simulink model "Simple_4Quad_payload_04"  (R2018b)
settings: Solver=VariableStepAuto  StartTime=0.0  StopTime=60  RelTol=1e-3
InitFcn:
  | Simple_4Quad_payload_04_const
values from neighbouring files (symbols this model uses):
  All_rho = [d1 0 0 ... (first row only)    [Colab_4Quad_model_01_const.m]    (also in Colab_4Quad_model_02_const.m; Simple_4Quad_payload_04_const.m; Simple_4Quad_payload_05_const.m; Simple_4Quad_payload_06_const.m)
  B_ob = [zeros(3);eye(3)]    [Simple_4Quad_payload_04_const.m]    (also in Simple_4Quad_payload_05_const.m; Simple_4Quad_payload_06_const.m; Simple_4Quad_payload_07_const.m; Simple_4Quad_payload_08_const.m)
  BBT_inv = ((B'*B)^(-1))*B'    [Simple_2Quad_payload_03_const.m]    (also in Simple_4Quad_payload_04_const.m = ((BR'*BR)^(-1))*BR'; Simple_4Quad_payload_05_const.m = ((BR'*BR)^(-1))*BR'; Simple_4Quad_payload_06_const.m = ((BR'*BR)^(-1))*BR'; Simple_4Quad_payload_07_const.m = ((BR'*BR)^(-1))*BR')
  BR = 1e0*eye(n)    [Simple_4Quad_payload_04_const.m]    (also in Simple_4Quad_payload_05_const.m; Simple_4Quad_payload_06_const.m; Simple_4Quad_payload_07_const.m; Simple_4Quad_payload_08_const.m)
  C_ob = [eye(3) zeros(3)]    [Simple_4Quad_payload_04_const.m]    (also in Simple_4Quad_payload_05_const.m; Simple_4Quad_payload_06_const.m; Simple_4Quad_payload_07_const.m; Simple_4Quad_payload_08_const.m)
  d1 = 0.25    [Colab_4Quad_model_01_const.m]    (also in Colab_4Quad_model_02_const.m = 0.5; Simple_4Quad_payload_01_const.m = 1; Simple_4Quad_payload_02_const.m = 1; Simple_4Quad_payload_03_const.m = 1)
  d2 = 0.25    [Colab_4Quad_model_01_const.m]    (also in Colab_4Quad_model_02_const.m = 0.5; Simple_4Quad_payload_01_const.m = 1; Simple_4Quad_payload_02_const.m = 1; Simple_4Quad_payload_03_const.m = 1)
  Des_rel_dist = 2    [Simple_4Quad_payload_01_const.m]    (also in Simple_4Quad_payload_02_const.m = 4; Simple_4Quad_payload_03_const.m = 4; Simple_4Quad_payload_04_const.m; Simple_4Quad_payload_05_const.m)
  g = 9.81    [Colab_4Quad_model_01_const.m]    (also in Colab_4Quad_model_02_const.m; Simple_2Quad_payload_01_const.m; Simple_2Quad_payload_02_const.m; Simple_2Quad_payload_03_const.m)
  gamma_0 = 1e-0*diag([1e-3;1e-0])    [Simple_2Quad_payload_03_const.m]    (also in Simple_4Quad_payload_04_const.m = 1e-0*diag([1e-6*ones(3,1);1e-0*ones(3,1)]); Simple_4Quad_payload_05_const.m = 1e-1*diag([1e-6*ones(3,1);1e-0*ones(3,1)]); Simple_4Quad_payload_06_const.m = 1e-0*diag([1e-6*ones(3,1);1e-0*ones(3,1)]); Simple_4Quad_payload_07_const.m = 1e-0*diag([1e-6*ones(3,1);1e-0*ones(3,1)]))
  gamma_1 = 1e+2*diag([1e-3;1e-0])    [Simple_2Quad_payload_03_const.m]    (also in Simple_4Quad_payload_04_const.m = 1e+2*diag([1e-6*ones(3,1);1e-0*ones(3,1)]); Simple_4Quad_payload_05_const.m = 1e+2*diag([1e-6*ones(3,1);1e-0*ones(3,1)]); Simple_4Quad_payload_06_const.m = 1e+3*diag([1e-6*ones(3,1);1e-0*ones(3,1)]); Simple_4Quad_payload_07_const.m = 1e+3*diag([1e-6*ones(3,1);1e-0*ones(3,1)]))
  Ix = 0.166667    [Colab_4Quad_model_01_const.m]    (also in Colab_4Quad_model_02_const.m = 0.02; Simple_4Quad_payload_01_const.m = 1; Simple_4Quad_payload_02_const.m = 1; Simple_4Quad_payload_03_const.m = 1)
  Iy = 0.166667    [Colab_4Quad_model_01_const.m]    (also in Colab_4Quad_model_02_const.m = 0.02; Simple_4Quad_payload_01_const.m = 1; Simple_4Quad_payload_02_const.m = 1; Simple_4Quad_payload_03_const.m = 1)
  Iz = 0.166667    [Colab_4Quad_model_01_const.m]    (also in Colab_4Quad_model_02_const.m = 0.02; Simple_4Quad_payload_01_const.m = 1; Simple_4Quad_payload_02_const.m = 1; Simple_4Quad_payload_03_const.m = 1)
  Jo = diag([Ix;Iy;Iz])    [Colab_4Quad_model_01_const.m]    (also in Colab_4Quad_model_02_const.m; Simple_4Quad_payload_04_const.m; Simple_4Quad_payload_05_const.m; Simple_4Quad_payload_06_const.m)
  Jq = diag([0.0291 0.0291 0.0552])    [Colab_4Quad_model_01_const.m]    (also in Colab_4Quad_model_02_const.m = diag([0.03 0.03 0.06]); Simple_4Quad_payload_03_const.m = 1.2416e-3 * diag([1 1 2]); Simple_4Quad_payload_04_const.m = 1 * diag([1 1 2]); Simple_4Quad_payload_05_const.m = 1 * diag([1 1 2]))
  k1 = 1    [Simple_2Quad_payload_03_const.m]    (also in Simple_4Quad_payload_04_const.m; Simple_4Quad_payload_05_const.m; Simple_4Quad_payload_06_const.m; Simple_4Quad_payload_07_const.m)
  k2 = 0.1    [Simple_2Quad_payload_03_const.m]    (also in Simple_4Quad_payload_04_const.m; Simple_4Quad_payload_05_const.m; Simple_4Quad_payload_06_const.m; Simple_4Quad_payload_07_const.m)
  ki1_N = 0    [Simple_4Quad_payload_02_const.m]    (also in Simple_4Quad_payload_03_const.m; Simple_4Quad_payload_04_const.m; Simple_4Quad_payload_05_const.m; Simple_4Quad_payload_06_const.m)
  ki1_S = 0    [Simple_4Quad_payload_02_const.m]    (also in Simple_4Quad_payload_03_const.m; Simple_4Quad_payload_04_const.m)
  ki2_N = 0    [Simple_4Quad_payload_02_const.m]    (also in Simple_4Quad_payload_03_const.m; Simple_4Quad_payload_04_const.m; Simple_4Quad_payload_05_const.m; Simple_4Quad_payload_06_const.m = 10)
  ki2_S = 0    [Simple_4Quad_payload_02_const.m]    (also in Simple_4Quad_payload_03_const.m; Simple_4Quad_payload_04_const.m)
  kp1_N = 10    [Simple_4Quad_payload_02_const.m]    (also in Simple_4Quad_payload_03_const.m; Simple_4Quad_payload_04_const.m; Simple_4Quad_payload_05_const.m = 1; Simple_4Quad_payload_06_const.m = 1)
  kp1_S = 10    [Simple_4Quad_payload_02_const.m]    (also in Simple_4Quad_payload_03_const.m; Simple_4Quad_payload_04_const.m)
  kp2_N = 100    [Simple_4Quad_payload_02_const.m]    (also in Simple_4Quad_payload_03_const.m; Simple_4Quad_payload_04_const.m; Simple_4Quad_payload_05_const.m = 1; Simple_4Quad_payload_06_const.m = 1)
  kp2_S = 100    [Simple_4Quad_payload_02_const.m]    (also in Simple_4Quad_payload_03_const.m; Simple_4Quad_payload_04_const.m)
  l = 3.1819    [Colab_4Quad_model_01_const.m]    (also in Colab_4Quad_model_02_const.m = 3; Simple_2Quad_payload_04_const.m = 1; Simple_4Quad_payload_01_const.m = 1; Simple_4Quad_payload_02_const.m = 2)
  m = 1.5    [Colab_4Quad_model_01_const.m]    (also in Colab_4Quad_model_02_const.m; Simple_2Quad_payload_04_const.m = 1; Simple_4Quad_payload_01_const.m = 1; Simple_4Quad_payload_02_const.m = 1)
  M = 1.0    (= 1)    [Colab_4Quad_model_01_const.m]    (also in Colab_4Quad_model_02_const.m; Simple_2Quad_payload_01_const.m; Simple_2Quad_payload_02_const.m; Simple_2Quad_payload_03_const.m)
  Md = 1*[1;1;1]    [Simple_2Quad_payload_04_const.m]    (also in Simple_4Quad_payload_01_const.m = 1*[1;1;1;1;1;1]; Simple_4Quad_payload_02_const.m = 1*[1;1;1;1;1;1]; Simple_4Quad_payload_03_const.m = 1*[1;1;1;1;1;1]; Simple_4Quad_payload_04_const.m = 1*[1;1;1;1;1;1])
  n = 2    [Simple_2Quad_payload_03_const.m]    (also in Simple_4Quad_payload_03_const.m = 6; Simple_4Quad_payload_04_const.m = 6; Simple_4Quad_payload_05_const.m = 6; Simple_4Quad_payload_06_const.m = 6)
  Q_ob = var_u_ob * eye(6)    [Simple_4Quad_payload_04_const.m]    (also in Simple_4Quad_payload_05_const.m; Simple_4Quad_payload_06_const.m; Simple_4Quad_payload_07_const.m; Simple_4Quad_payload_08_const.m)
  QR = 1e-0*eye(n)    [Simple_4Quad_payload_04_const.m]    (also in Simple_4Quad_payload_05_const.m = 1e-1*eye(n); Simple_4Quad_payload_06_const.m; Simple_4Quad_payload_07_const.m; Simple_4Quad_payload_08_const.m)
  R = 1e+0*eye(n)    [Simple_2Quad_payload_03_const.m]    (also in Simple_4Quad_payload_04_const.m = 1e+0*eye(m); Simple_4Quad_payload_05_const.m = 1e+0*eye(m); Simple_4Quad_payload_06_const.m; Simple_4Quad_payload_07_const.m)
  R_ob = var_y_ob * eye(3)    [Simple_4Quad_payload_04_const.m]    (also in Simple_4Quad_payload_05_const.m; Simple_4Quad_payload_06_const.m; Simple_4Quad_payload_07_const.m; Simple_4Quad_payload_08_const.m)
  rho_0 = 1e-0    (= 1)    [Simple_2Quad_payload_03_const.m]    (also in Simple_4Quad_payload_04_const.m; Simple_4Quad_payload_05_const.m = 0.1; Simple_4Quad_payload_06_const.m; Simple_4Quad_payload_07_const.m)
  rho_1 = 1e-0    (= 1)    [Simple_2Quad_payload_03_const.m]    (also in Simple_4Quad_payload_04_const.m; Simple_4Quad_payload_05_const.m; Simple_4Quad_payload_06_const.m; Simple_4Quad_payload_07_const.m)
libraries: simulink x16
(part 1 of 4)
settings Model: Creator=ali  LastModifiedBy=asafae

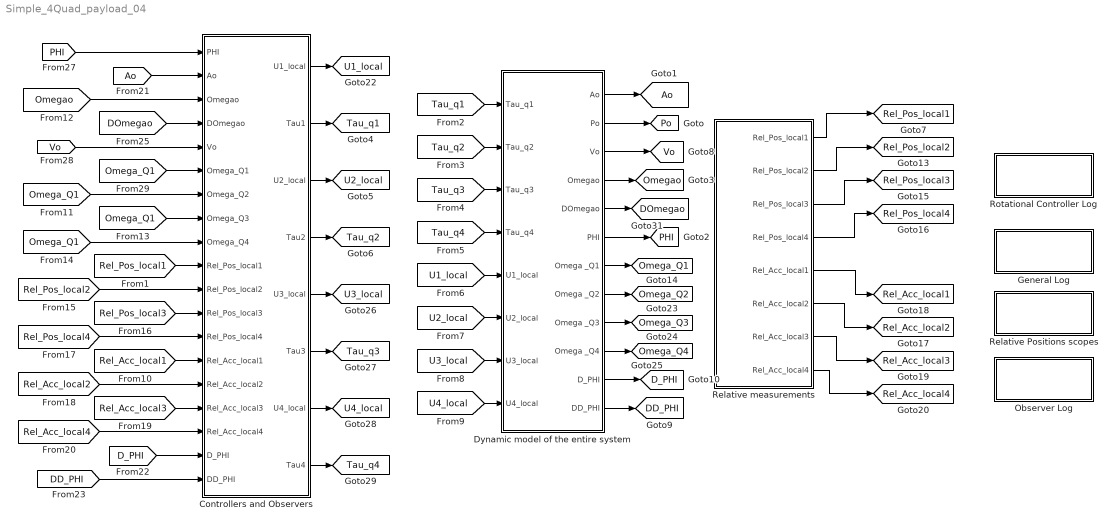
== system Simple_4Quad_payload_04 ==
  Controllers and Observers : Subsystem
  Dynamic model of the entire system : Subsystem
  General Log : Subsystem
  Observer Log : Subsystem
  Relative Positions scopes : Subsystem
  Relative measurements : Subsystem
  Rotational Controller Log : Subsystem
  tag scope: Ao=global, DD_PHI=global, DOmegao=global, D_PHI=global, Omega_Q1=global, Omega_Q2=global, Omega_Q3=global, Omega_Q4=global, Omegao=global, PHI=global, Po=global, Rel_Acc_local1=global, Rel_Acc_local2=global, Rel_Acc_local3=global, Rel_Acc_local4=global, Rel_Pos_local1=global, Rel_Pos_local2=global, Rel_Pos_local3=global, Rel_Pos_local4=global, Tau_q1=global, Tau_q2=global, Tau_q3=global, Tau_q4=global, U1_local=global, U2_local=global, U3_local=global, U4_local=global, Vo=global
  wires:
  [Tau_q1] -> Dynamic model of the entire system/1(Tau_q1)
  [Tau_q2] -> Dynamic model of the entire system/2(Tau_q2)
  [Tau_q3] -> Dynamic model of the entire system/3(Tau_q3)
  [Tau_q4] -> Dynamic model of the entire system/4(Tau_q4)
  [U1_local] -> Dynamic model of the entire system/5(U1_local)
  [U2_local] -> Dynamic model of the entire system/6(U2_local)
  [U3_local] -> Dynamic model of the entire system/7(U3_local)
  [U4_local] -> Dynamic model of the entire system/8(U4_local)
  Dynamic model of the entire system/6(PHI) -> [PHI]
  Dynamic model of the entire system/4(Omegao) -> [Omegao]
  Dynamic model of the entire system/1(Ao) -> [Ao]
  Dynamic model of the entire system/2(Po) -> [Po]
  Dynamic model of the entire system/5(DOmegao) -> [DOmegao]
  Dynamic model of the entire system/7(Omega _Q1) -> [Omega_Q1]
  Dynamic model of the entire system/8(Omega _Q2) -> [Omega_Q2]
  Dynamic model of the entire system/9(Omega _Q3) -> [Omega_Q3]
  Dynamic model of the entire system/10(Omega _Q4) -> [Omega_Q4]
  Controllers and Observers/1(U1_local) -> [U1_local]
  Controllers and Observers/2(Tau1) -> [Tau_q1]
  Controllers and Observers/3(U2_local) -> [U2_local]
  Controllers and Observers/4(Tau2) -> [Tau_q2]
  Controllers and Observers/8(Tau4) -> [Tau_q4]
  Controllers and Observers/7(U4_local) -> [U4_local]
  Controllers and Observers/6(Tau3) -> [Tau_q3]
  Controllers and Observers/5(U3_local) -> [U3_local]
  [Omegao] -> Controllers and Observers/3(Omegao)
  [DOmegao] -> Controllers and Observers/4(DOmegao)
  [Omega_Q1] -> Controllers and Observers/6(Omega_Q1)
  [Omega_Q1] -> Controllers and Observers/7(Omega_Q2)
  [Omega_Q1] -> Controllers and Observers/8(Omega_Q3)
  [Omega_Q1] -> Controllers and Observers/9(Omega_Q4)
  [Rel_Pos_local1] -> Controllers and Observers/10(Rel_Pos_local1)
  [Rel_Pos_local2] -> Controllers and Observers/11(Rel_Pos_local2)
  [Rel_Pos_local3] -> Controllers and Observers/12(Rel_Pos_local3)
  [Rel_Pos_local4] -> Controllers and Observers/13(Rel_Pos_local4)
  [Rel_Acc_local1] -> Controllers and Observers/14(Rel_Acc_local1)
  [Rel_Acc_local2] -> Controllers and Observers/15(Rel_Acc_local2)
  [Rel_Acc_local3] -> Controllers and Observers/16(Rel_Acc_local3)
  [Rel_Acc_local4] -> Controllers and Observers/17(Rel_Acc_local4)
  Relative measurements/1(Rel_Pos_local1) -> [Rel_Pos_local1]
  Relative measurements/2(Rel_Pos_local2) -> [Rel_Pos_local2]
  Relative measurements/3(Rel_Pos_local3) -> [Rel_Pos_local3]
  Relative measurements/4(Rel_Pos_local4) -> [Rel_Pos_local4]
  Relative measurements/5(Rel_Acc_local1) -> [Rel_Acc_local1]
  Relative measurements/6(Rel_Acc_local2) -> [Rel_Acc_local2]
  Relative measurements/7(Rel_Acc_local3) -> [Rel_Acc_local3]
  Relative measurements/8(Rel_Acc_local4) -> [Rel_Acc_local4]
  Dynamic model of the entire system/3(Vo) -> [Vo]
  [Vo] -> Controllers and Observers/5(Vo)
  [PHI] -> Controllers and Observers/1(PHI)
  [Ao] -> Controllers and Observers/2(Ao)
  Dynamic model of the entire system/11(D_PHI) -> [D_PHI]
  Dynamic model of the entire system/12(DD_PHI) -> [DD_PHI]
  [D_PHI] -> Controllers and Observers/18(D_PHI)
  [DD_PHI] -> Controllers and Observers/19(DD_PHI)

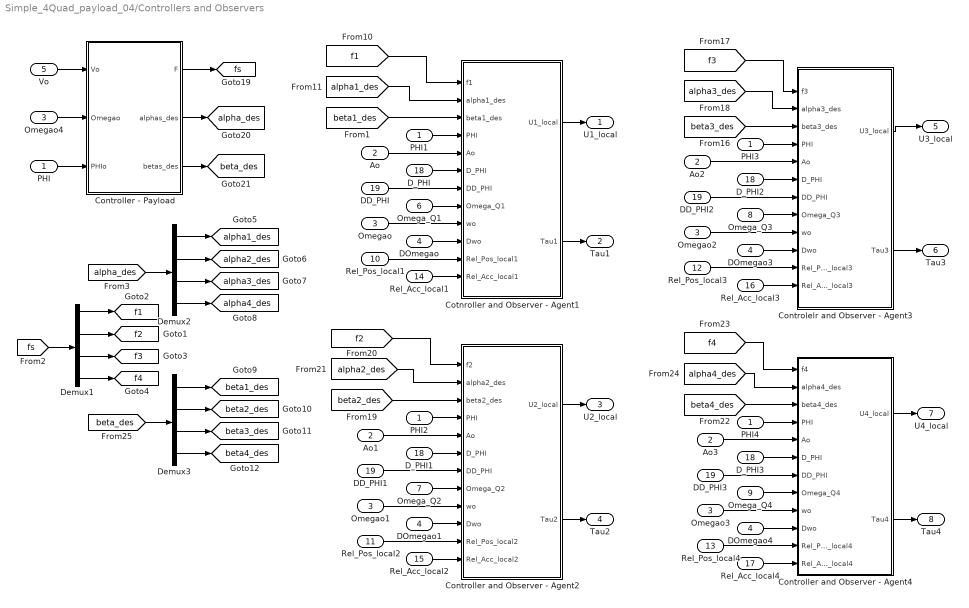
== system Simple_4Quad_payload_04/Controllers and Observers ==
  PHI : Inport
  Ao : Inport  Port=2
  Omegao : Inport  Port=3
  DOmegao : Inport  Port=4
  Vo : Inport  Port=5
  Omega_Q1 : Inport  Port=6
  Omega_Q2 : Inport  Port=7
  Omega_Q3 : Inport  Port=8
  Omega_Q4 : Inport  Port=9
  Rel_Pos_local1 : Inport  Port=10
  Rel_Pos_local2 : Inport  Port=11
  Rel_Pos_local3 : Inport  Port=12
  Rel_Pos_local4 : Inport  Port=13
  Rel_Acc_local1 : Inport  Port=14
  Rel_Acc_local2 : Inport  Port=15
  Rel_Acc_local3 : Inport  Port=16
  Rel_Acc_local4 : Inport  Port=17
  D_PHI : Inport  Port=18
  DD_PHI : Inport  Port=19
  Ao1 : InportShadow  Port=2
  Ao2 : InportShadow  Port=2
  Ao3 : InportShadow  Port=2
  Controlelr and Observer - Agent3 : Subsystem
  Controller - Payload : Subsystem
  Controller and Observer - Agent2 : Subsystem
  Controller and Observer - Agent4 : Subsystem
  "Cotnroller and Observer - Agent1 " : Subsystem
  DD_PHI1 : InportShadow  Port=19
  DD_PHI2 : InportShadow  Port=19
  DD_PHI3 : InportShadow  Port=19
  DOmegao1 : InportShadow  Port=4
  DOmegao3 : InportShadow  Port=4
  DOmegao4 : InportShadow  Port=4
  D_PHI1 : InportShadow  Port=18
  D_PHI2 : InportShadow  Port=18
  D_PHI3 : InportShadow  Port=18
  Demux1 : Demux
  Demux2 : Demux
  Demux3 : Demux
  Omegao{1..4} (4 alike) : InportShadow  Port=3
  PHI{1..4} (4 alike) : InportShadow
  U1_local : Outport
  Tau1 : Outport  Port=2
  U2_local : Outport  Port=3
  Tau2 : Outport  Port=4
  U3_local : Outport  Port=5
  Tau3 : Outport  Port=6
  U4_local : Outport  Port=7
  Tau4 : Outport  Port=8
  tag scope: alpha1_des=global, alpha2_des=global, alpha3_des=global, alpha4_des=global, alpha_des=global, beta1_des=global, beta2_des=global, beta3_des=global, beta4_des=global, beta_des=global, f1=global, f2=global, f3=global, f4=global, fs=global
  wires:
  Controller and Observer - Agent4/2(Tau4) -> Tau4/1
  Controller and Observer - Agent4/1(U4_local) -> U4_local/1
  Controlelr and Observer - Agent3/2(Tau3) -> Tau3/1
  Controlelr and Observer - Agent3/1(U3_local) -> U3_local/1
  Controller and Observer - Agent2/1(U2_local) -> U2_local/1
  "Cotnroller and Observer - Agent1 "/1(U1_local) -> U1_local/1
  Controller and Observer - Agent2/2(Tau2) -> Tau2/1
  Omega_Q1/1 -> "Cotnroller and Observer - Agent1 "/8(Omega_Q1)
  Omega_Q3/1 -> Controlelr and Observer - Agent3/8(Omega_Q3)
  Omega_Q4/1 -> Controller and Observer - Agent4/8(Omega_Q4)
  Omega_Q2/1 -> Controller and Observer - Agent2/8(Omega_Q2)
  "Cotnroller and Observer - Agent1 "/2(Tau1) -> Tau1/1
  [f1] -> "Cotnroller and Observer - Agent1 "/1(f1)
  Controller - Payload/2(alphas_des) -> [alpha_des]
  Vo/1 -> Controller - Payload/1(Vo)
  Omegao4/1 -> Controller - Payload/2(Omegao)
  PHI/1 -> Controller - Payload/3(PHIo)
  Controller - Payload/1(F) -> [fs]
  Controller - Payload/3(betas_des) -> [beta_des]
  [beta1_des] -> "Cotnroller and Observer - Agent1 "/3(beta1_des)
  [alpha1_des] -> "Cotnroller and Observer - Agent1 "/2(alpha1_des)
  Rel_Pos_local1/1 -> "Cotnroller and Observer - Agent1 "/11(Rel_Pos_local1)
  Rel_Acc_local1/1 -> "Cotnroller and Observer - Agent1 "/12(Rel_Acc_local1)
  Rel_Pos_local2/1 -> Controller and Observer - Agent2/11(Rel_Pos_local2)
  Rel_Acc_local2/1 -> Controller and Observer - Agent2/12(Rel_Acc_local2)
  Rel_Pos_local4/1 -> Controller and Observer - Agent4/11(Rel_Pos_local4)
  Rel_Acc_local4/1 -> Controller and Observer - Agent4/12(Rel_Acc_local4)
  Rel_Pos_local3/1 -> Controlelr and Observer - Agent3/11(Rel_Pos_local3)
  Rel_Acc_local3/1 -> Controlelr and Observer - Agent3/12(Rel_Acc_local3)
  [f3] -> Controlelr and Observer - Agent3/1(f3)
  [alpha3_des] -> Controlelr and Observer - Agent3/2(alpha3_des)
  [beta3_des] -> Controlelr and Observer - Agent3/3(beta3_des)
  [f2] -> Controller and Observer - Agent2/1(f2)
  [alpha2_des] -> Controller and Observer - Agent2/2(alpha2_des)
  [beta2_des] -> Controller and Observer - Agent2/3(beta2_des)
  [f4] -> Controller and Observer - Agent4/1(f4)
  [alpha4_des] -> Controller and Observer - Agent4/2(alpha4_des)
  [beta4_des] -> Controller and Observer - Agent4/3(beta4_des)
  DOmegao/1 -> "Cotnroller and Observer - Agent1 "/10(Dwo)
  DOmegao1/1 -> Controller and Observer - Agent2/10(Dwo)
  DOmegao3/1 -> Controlelr and Observer - Agent3/10(Dwo)
  DOmegao4/1 -> Controller and Observer - Agent4/10(Dwo)
  Omegao/1 -> "Cotnroller and Observer - Agent1 "/9(wo)
  Omegao2/1 -> Controlelr and Observer - Agent3/9(wo)
  Omegao1/1 -> Controller and Observer - Agent2/9(wo)
  Omegao3/1 -> Controller and Observer - Agent4/9(wo)
  Demux2/2 -> [alpha2_des]
  Demux3/3 -> [beta3_des]
  Demux2/4 -> [alpha4_des]
  Demux2/3 -> [alpha3_des]
  Demux1/4 -> [f4]
  Demux2/1 -> [alpha1_des]
  Demux1/1 -> [f1]
  [alpha_des] -> Demux2/1
  Demux3/4 -> [beta4_des]
  [beta_des] -> Demux3/1
  [fs] -> Demux1/1
  Demux3/2 -> [beta2_des]
  Demux1/3 -> [f3]
  Demux1/2 -> [f2]
  Demux3/1 -> [beta1_des]
  PHI1/1 -> "Cotnroller and Observer - Agent1 "/4(PHI)
  Ao/1 -> "Cotnroller and Observer - Agent1 "/5(Ao)
  PHI2/1 -> Controller and Observer - Agent2/4(PHI)
  Ao1/1 -> Controller and Observer - Agent2/5(Ao)
  PHI3/1 -> Controlelr and Observer - Agent3/4(PHI)
  Ao2/1 -> Controlelr and Observer - Agent3/5(Ao)
  PHI4/1 -> Controller and Observer - Agent4/4(PHI)
  Ao3/1 -> Controller and Observer - Agent4/5(Ao)
  D_PHI/1 -> "Cotnroller and Observer - Agent1 "/6(D_PHI)
  DD_PHI/1 -> "Cotnroller and Observer - Agent1 "/7(DD_PHI)
  DD_PHI1/1 -> Controller and Observer - Agent2/7(DD_PHI)
  D_PHI1/1 -> Controller and Observer - Agent2/6(D_PHI)
  D_PHI2/1 -> Controlelr and Observer - Agent3/6(D_PHI)
  DD_PHI2/1 -> Controlelr and Observer - Agent3/7(DD_PHI)
  D_PHI3/1 -> Controller and Observer - Agent4/6(D_PHI)
  DD_PHI3/1 -> Controller and Observer - Agent4/7(DD_PHI)

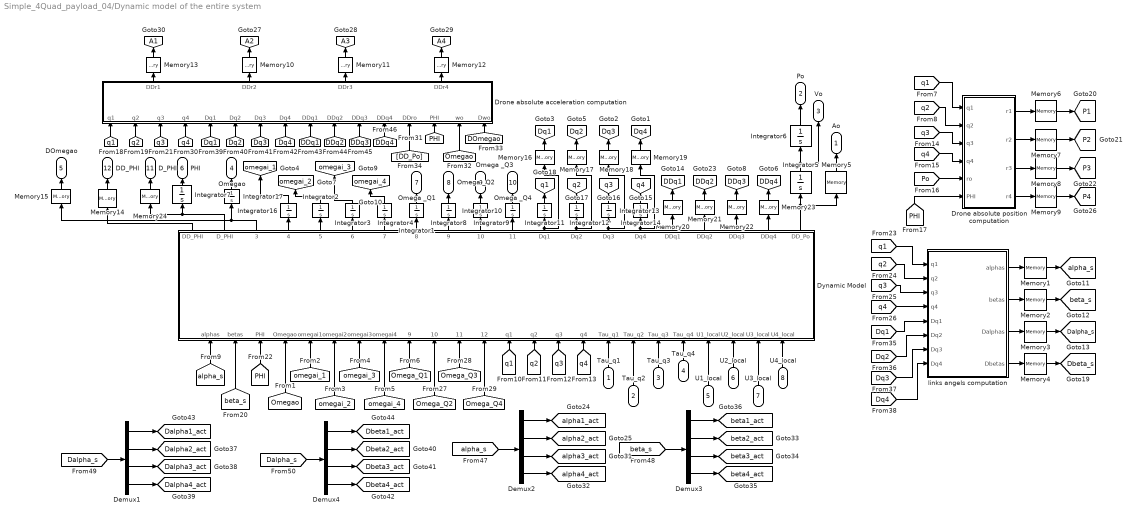
== system Simple_4Quad_payload_04/Dynamic model of the entire system ==
  Tau_q1 : Inport
  Tau_q2 : Inport  Port=2
  Tau_q3 : Inport  Port=3
  Tau_q4 : Inport  Port=4
  U1_local : Inport  Port=5
  U2_local : Inport  Port=6
  U3_local : Inport  Port=7
  U4_local : Inport  Port=8
  Demux{1..4} (4 alike) : Demux
  Drone absolute acceleration computation : MATLAB Function  TreatAsAtomicUnit=on
  Drone absolute position computation : MATLAB Function  TreatAsAtomicUnit=on
  "Dynamic Model " : MATLAB Function  TreatAsAtomicUnit=on
  Integrator{1..5,7..10,16..17} (11 alike) : Integrator  InitialCondition=zeros(3,1)
  Integrator{11..14} (4 alike) : Integrator  InitialCondition=[0;0;1]
  Integrator6 : Integrator  InitialCondition=[0;0;0]
  Memory1 : Memory  InitialCondition=pi/2*ones(4,1)
  Memory{5,10..24} (16 alike) : Memory  InitialCondition=zeros(3,1)
  Memory2 : Memory  InitialCondition=zeros(4,1)
  Memory3 : Memory  InitialCondition=zeros(4,1)
  Memory4 : Memory  InitialCondition=zeros(4,1)
  Memory6 : Memory  InitialCondition=[d1;0;l]
  Memory7 : Memory  InitialCondition=[-d1;0;l]
  Memory8 : Memory  InitialCondition=[0;d2;l]
  Memory9 : Memory  InitialCondition=[0;-d2;l]
  links angels computation : MATLAB Function  TreatAsAtomicUnit=on
  Ao : Outport
  Po : Outport  Port=2
  Vo : Outport  Port=3
  Omegao : Outport  Port=4
  DOmegao : Outport  Port=5
  PHI : Outport  Port=6
  Omega _Q1 : Outport  Port=7
  Omega _Q2 : Outport  Port=8
  Omega _Q3 : Outport  Port=9
  Omega _Q4 : Outport  Port=10
  D_PHI : Outport  Port=11
  DD_PHI : Outport  Port=12
  tag scope: A1=global, A2=global, A3=global, A4=global, DDq1=global, DDq2=global, DDq3=global, DDq4=global, Dalpha1_act=global, Dalpha2_act=global, Dalpha3_act=global, Dalpha4_act=global, Dalpha_s=global, Dbeta1_act=global, Dbeta2_act=global, Dbeta3_act=global, Dbeta4_act=global, Dbeta_s=global, Dq1=global, Dq2=global, Dq3=global, Dq4=global, P1=global, P2=global, P3=global, P4=global, alpha1_act=global, alpha2_act=global, alpha3_act=global, alpha4_act=global, alpha_s=global, beta1_act=global, beta2_act=global, beta3_act=global, beta4_act=global, beta_s=global, omegai_1=global, omegai_2=global, omegai_3=global, omegai_4=global, q1=global, q2=global, q3=global, q4=global
  wires:
  links angels computation/1(alphas) -> Memory1/1
  links angels computation/2(betas) -> Memory2/1
  links angels computation/3(Dalphas) -> Memory3/1
  links angels computation/4(Dbetas) -> Memory4/1
  Integrator5/1 -> Vo/1, Integrator6/1
  Integrator1/1 -> Omega _Q1/1
  Integrator2/1 -> [omegai_2]
  Integrator3/1 -> [omegai_3]
  Integrator6/1 -> Po/1
  Integrator4/1 -> [omegai_4]
  Memory5/1 -> Ao/1
  Integrator17/1 -> Omegao/1
  Integrator7/1 -> PHI/1
  [q1] -> links angels computation/1(q1)
  [q2] -> links angels computation/2(q2)
  [q3] -> links angels computation/3(q3)
  [q4] -> links angels computation/4(q4)
  "Dynamic Model "/20(DD_Po) -> Memory5/1, Integrator5/1
  "Dynamic Model "/2(D_PHI) -> Memory24/1, Integrator7/1
  "Dynamic Model "/1(DD_PHI) -> Memory14/1
  "Dynamic Model "/7(D_omegai_4) -> Integrator4/1
  "Dynamic Model "/6(D_omegai_3) -> Integrator3/1
  "Dynamic Model "/5(D_omegai_2) -> Integrator2/1
  "Dynamic Model "/4(D_omegai_1) -> Integrator16/1
  "Dynamic Model "/3(D_Omegao) -> Memory15/1, Integrator17/1
  Integrator16/1 -> [omegai_1]
  "Dynamic Model "/8(D_Omega_Q1) -> Integrator1/1
  "Dynamic Model "/9(D_Omega_Q2) -> Integrator8/1
  "Dynamic Model "/10(D_Omega_Q3) -> Integrator9/1
  "Dynamic Model "/11(D_Omega_Q4) -> Integrator10/1
  Integrator8/1 -> Omega _Q2/1
  Integrator10/1 -> Omega _Q4/1
  Integrator9/1 -> Omega _Q3/1
  "Dynamic Model "/12(Dq1) -> Memory16/1, Integrator11/1
  "Dynamic Model "/13(Dq2) -> Memory17/1, Integrator12/1
  "Dynamic Model "/14(Dq3) -> Memory18/1, Integrator13/1
  "Dynamic Model "/15(Dq4) -> Memory19/1, Integrator14/1
  Integrator14/1 -> [q4]
  Integrator13/1 -> [q3]
  Integrator12/1 -> [q2]
  Integrator11/1 -> [q1]
  [PHI] -> "Dynamic Model "/3(PHI)
  [Omegao] -> "Dynamic Model "/4(Omegao)
  [omegai_1] -> "Dynamic Model "/5(omegai1)
  [omegai_2] -> "Dynamic Model "/6(omegai2)
  [omegai_3] -> "Dynamic Model "/7(omegai3)
  [omegai_4] -> "Dynamic Model "/8(omegai4)
  [Omega_Q1] -> "Dynamic Model "/9(Omega_q1)
  [Omega_Q2] -> "Dynamic Model "/10(Omega_q2)
  [Omega_Q3] -> "Dynamic Model "/11(Omega_q3)
  [Omega_Q4] -> "Dynamic Model "/12(Omega_q4)
  [q1] -> "Dynamic Model "/13(q1)
  [q2] -> "Dynamic Model "/14(q2)
  [q3] -> "Dynamic Model "/15(q3)
  [q4] -> "Dynamic Model "/16(q4)
  Tau_q2/1 -> "Dynamic Model "/18(Tau_q2)
  Tau_q4/1 -> "Dynamic Model "/20(Tau_q4)
  U2_local/1 -> "Dynamic Model "/22(U2_local)
  U4_local/1 -> "Dynamic Model "/24(U4_local)
  [beta_s] -> "Dynamic Model "/2(betas)
  [alpha_s] -> "Dynamic Model "/1(alphas)
  Tau_q1/1 -> "Dynamic Model "/17(Tau_q1)
  Tau_q3/1 -> "Dynamic Model "/19(Tau_q3)
  U1_local/1 -> "Dynamic Model "/21(U1_local)
  U3_local/1 -> "Dynamic Model "/23(U3_local)
  Memory4/1 -> [Dbeta_s]
  Memory2/1 -> [beta_s]
  Memory3/1 -> [Dalpha_s]
  Memory1/1 -> [alpha_s]
  [q1] -> Drone absolute position computation/1(q1)
  [q2] -> Drone absolute position computation/2(q2)
  [q3] -> Drone absolute position computation/3(q3)
  [q4] -> Drone absolute position computation/4(q4)
  [Po] -> Drone absolute position computation/5(ro)
  [PHI] -> Drone absolute position computation/6(PHI)
  Memory6/1 -> [P1]
  Memory8/1 -> [P3]
  Memory7/1 -> [P2]
  Memory9/1 -> [P4]
  Drone absolute position computation/4(r4) -> Memory9/1
  Drone absolute position computation/3(r3) -> Memory8/1
  Drone absolute position computation/2(r2) -> Memory7/1
  Drone absolute position computation/1(r1) -> Memory6/1
  [q1] -> Drone absolute acceleration computation/1(q1)
  [q2] -> Drone absolute acceleration computation/2(q2)
  [q3] -> Drone absolute acceleration computation/3(q3)
  [q4] -> Drone absolute acceleration computation/4(q4)
  [PHI] -> Drone absolute acceleration computation/14(PHI)
  [Omegao] -> Drone absolute acceleration computation/15(wo)
  Memory13/1 -> [A1]
  Drone absolute acceleration computation/1(DDr1) -> Memory13/1
  Memory10/1 -> [A2]
  Drone absolute acceleration computation/2(DDr2) -> Memory10/1
  Memory11/1 -> [A3]
  Drone absolute acceleration computation/3(DDr3) -> Memory11/1
  Memory12/1 -> [A4]
  Drone absolute acceleration computation/4(DDr4) -> Memory12/1
  Memory14/1 -> DD_PHI/1
  Memory15/1 -> DOmegao/1
  [DOmegao] -> Drone absolute acceleration computation/16(Dwo)
  [DD_Po] -> Drone absolute acceleration computation/13(DDro)
  [Dq1] -> links angels computation/5(Dq1)
  [Dq2] -> links angels computation/6(Dq2)
  [Dq3] -> links angels computation/7(Dq3)
  [Dq4] -> links angels computation/8(Dq4)
  Memory19/1 -> [Dq4]
  Memory18/1 -> [Dq3]
  Memory16/1 -> [Dq1]
  Memory17/1 -> [Dq2]
  [Dq4] -> Drone absolute acceleration computation/8(Dq4)
  [Dq3] -> Drone absolute acceleration computation/7(Dq3)
  [Dq2] -> Drone absolute acceleration computation/6(Dq2)
  [Dq1] -> Drone absolute acceleration computation/5(Dq1)
  Memory21/1 -> [DDq2]
  Memory20/1 -> [DDq1]
  Memory22/1 -> [DDq3]
  Memory23/1 -> [DDq4]
  "Dynamic Model "/16(DDq1) -> Memory20/1
  "Dynamic Model "/17(DDq2) -> Memory21/1
  "Dynamic Model "/18(DDq3) -> Memory22/1
  "Dynamic Model "/19(DDq4) -> Memory23/1
  [DDq1] -> Drone absolute acceleration computation/9(DDq1)
  [DDq2] -> Drone absolute acceleration computation/10(DDq2)
  [DDq3] -> Drone absolute acceleration computation/11(DDq3)
  [DDq4] -> Drone absolute acceleration computation/12(DDq4)
  Memory24/1 -> D_PHI/1
  [alpha_s] -> Demux2/1
  Demux2/2 -> [alpha2_act]
  Demux2/3 -> [alpha3_act]
  Demux2/4 -> [alpha4_act]
  Demux2/1 -> [alpha1_act]
  Demux3/1 -> [beta1_act]
  [beta_s] -> Demux3/1
  Demux3/4 -> [beta4_act]
  Demux3/2 -> [beta2_act]
  Demux3/3 -> [beta3_act]
  Demux1/2 -> [Dalpha2_act]
  Demux1/1 -> [Dalpha1_act]
  Demux1/4 -> [Dalpha4_act]
  Demux4/4 -> [Dbeta4_act]
  [Dalpha_s] -> Demux1/1
  Demux4/3 -> [Dbeta3_act]
  Demux4/2 -> [Dbeta2_act]
  Demux4/1 -> [Dbeta1_act]
  Demux1/3 -> [Dalpha3_act]
  [Dalpha_s] -> Demux4/1

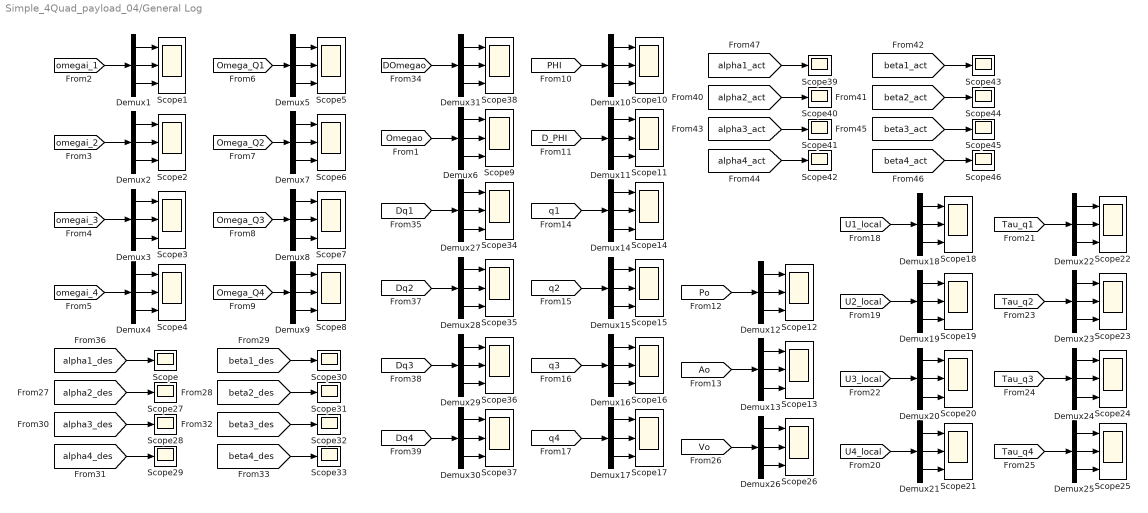
== system Simple_4Quad_payload_04/General Log ==
  Demux{1..31} (31 alike) : Demux  Outputs=3
  Scope{,27..33,39..46} (16 alike) : Scope
  Scope{1..26,34..38} (31 alike) : Scope  NumInputPorts=3
  wires:
  Demux6/2 -> Scope9/2
  Demux6/1 -> Scope9/1
  Demux6/3 -> Scope9/3
  [Omegao] -> Demux6/1
  [omegai_1] -> Demux1/1
  Demux1/3 -> Scope1/3
  Demux1/1 -> Scope1/1
  Demux1/2 -> Scope1/2
  Demux2/2 -> Scope2/2
  Demux2/1 -> Scope2/1
  Demux2/3 -> Scope2/3
  [omegai_2] -> Demux2/1
  [omegai_3] -> Demux3/1
  Demux3/3 -> Scope3/3
  Demux3/1 -> Scope3/1
  Demux3/2 -> Scope3/2
  Demux4/2 -> Scope4/2
  Demux4/1 -> Scope4/1
  Demux4/3 -> Scope4/3
  [omegai_4] -> Demux4/1
  [Omega_Q4] -> Demux9/1
  Demux9/3 -> Scope8/3
  Demux9/1 -> Scope8/1
  Demux9/2 -> Scope8/2
  Demux8/2 -> Scope7/2
  Demux8/1 -> Scope7/1
  Demux8/3 -> Scope7/3
  [Omega_Q3] -> Demux8/1
  [Omega_Q2] -> Demux7/1
  Demux7/3 -> Scope6/3
  Demux7/1 -> Scope6/1
  Demux7/2 -> Scope6/2
  Demux5/2 -> Scope5/2
  Demux5/1 -> Scope5/1
  Demux5/3 -> Scope5/3
  [Omega_Q1] -> Demux5/1
  [PHI] -> Demux10/1
  Demux10/3 -> Scope10/3
  Demux10/1 -> Scope10/1
  Demux10/2 -> Scope10/2
  Demux11/2 -> Scope11/2
  Demux11/1 -> Scope11/1
  Demux11/3 -> Scope11/3
  [D_PHI] -> Demux11/1
  [Po] -> Demux12/1
  Demux12/3 -> Scope12/3
  Demux12/1 -> Scope12/1
  Demux12/2 -> Scope12/2
  Demux13/2 -> Scope13/2
  Demux13/1 -> Scope13/1
  Demux13/3 -> Scope13/3
  [Ao] -> Demux13/1
  [q4] -> Demux17/1
  Demux17/3 -> Scope17/3
  Demux17/1 -> Scope17/1
  Demux17/2 -> Scope17/2
  Demux16/2 -> Scope16/2
  Demux16/1 -> Scope16/1
  Demux16/3 -> Scope16/3
  [q3] -> Demux16/1
  [q2] -> Demux15/1
  Demux15/3 -> Scope15/3
  Demux15/1 -> Scope15/1
  Demux15/2 -> Scope15/2
  Demux14/2 -> Scope14/2
  Demux14/1 -> Scope14/1
  Demux14/3 -> Scope14/3
  [q1] -> Demux14/1
  [U1_local] -> Demux18/1
  Demux18/3 -> Scope18/3
  Demux18/1 -> Scope18/1
  Demux18/2 -> Scope18/2
  Demux19/2 -> Scope19/2
  Demux19/1 -> Scope19/1
  Demux19/3 -> Scope19/3
  [U2_local] -> Demux19/1
  [U3_local] -> Demux20/1
  Demux20/3 -> Scope20/3
  Demux20/1 -> Scope20/1
  Demux20/2 -> Scope20/2
  Demux21/2 -> Scope21/2
  Demux21/1 -> Scope21/1
  Demux21/3 -> Scope21/3
  [U4_local] -> Demux21/1
  [Tau_q4] -> Demux25/1
  Demux25/3 -> Scope25/3
  Demux25/1 -> Scope25/1
  Demux25/2 -> Scope25/2
  Demux24/2 -> Scope24/2
  Demux24/1 -> Scope24/1
  Demux24/3 -> Scope24/3
  [Tau_q3] -> Demux24/1
  [Tau_q2] -> Demux23/1
  Demux23/3 -> Scope23/3
  Demux23/1 -> Scope23/1
  Demux23/2 -> Scope23/2
  Demux22/2 -> Scope22/2
  Demux22/1 -> Scope22/1
  Demux22/3 -> Scope22/3
  [Tau_q1] -> Demux22/1
  [Vo] -> Demux26/1
  Demux26/3 -> Scope26/3
  Demux26/1 -> Scope26/1
  Demux26/2 -> Scope26/2
  [alpha1_des] -> Scope/1
  [alpha3_des] -> Scope28/1
  [alpha2_des] -> Scope27/1
  [beta4_des] -> Scope33/1
  [beta1_des] -> Scope30/1
  [beta2_des] -> Scope31/1
  [alpha4_des] -> Scope29/1
  [beta3_des] -> Scope32/1
  [DOmegao] -> Demux31/1
  Demux31/3 -> Scope38/3
  Demux31/1 -> Scope38/1
  Demux31/2 -> Scope38/2
  [Dq1] -> Demux27/1
  Demux27/3 -> Scope34/3
  Demux27/1 -> Scope34/1
  Demux27/2 -> Scope34/2
  Demux28/2 -> Scope35/2
  Demux28/1 -> Scope35/1
  Demux28/3 -> Scope35/3
  [Dq2] -> Demux28/1
  [Dq3] -> Demux29/1
  Demux29/3 -> Scope36/3
  Demux29/1 -> Scope36/1
  Demux29/2 -> Scope36/2
  Demux30/2 -> Scope37/2
  Demux30/1 -> Scope37/1
  Demux30/3 -> Scope37/3
  [Dq4] -> Demux30/1
  [beta3_act] -> Scope45/1
  [alpha1_act] -> Scope39/1
  [beta4_act] -> Scope46/1
  [alpha3_act] -> Scope41/1
  [beta1_act] -> Scope43/1
  [beta2_act] -> Scope44/1
  [alpha4_act] -> Scope42/1
  [alpha2_act] -> Scope40/1

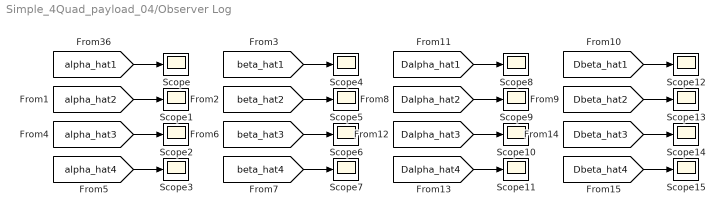
== system Simple_4Quad_payload_04/Observer Log ==
  Scope{,1..15} (16 alike) : Scope
  wires:
  [alpha_hat1] -> Scope/1
  [alpha_hat2] -> Scope1/1
  [alpha_hat3] -> Scope2/1
  [alpha_hat4] -> Scope3/1
  [beta_hat4] -> Scope7/1
  [beta_hat3] -> Scope6/1
  [beta_hat2] -> Scope5/1
  [beta_hat1] -> Scope4/1
  [Dbeta_hat1] -> Scope12/1
  [Dbeta_hat2] -> Scope13/1
  [Dbeta_hat3] -> Scope14/1
  [Dbeta_hat4] -> Scope15/1
  [Dalpha_hat4] -> Scope11/1
  [Dalpha_hat3] -> Scope10/1
  [Dalpha_hat2] -> Scope9/1
  [Dalpha_hat1] -> Scope8/1

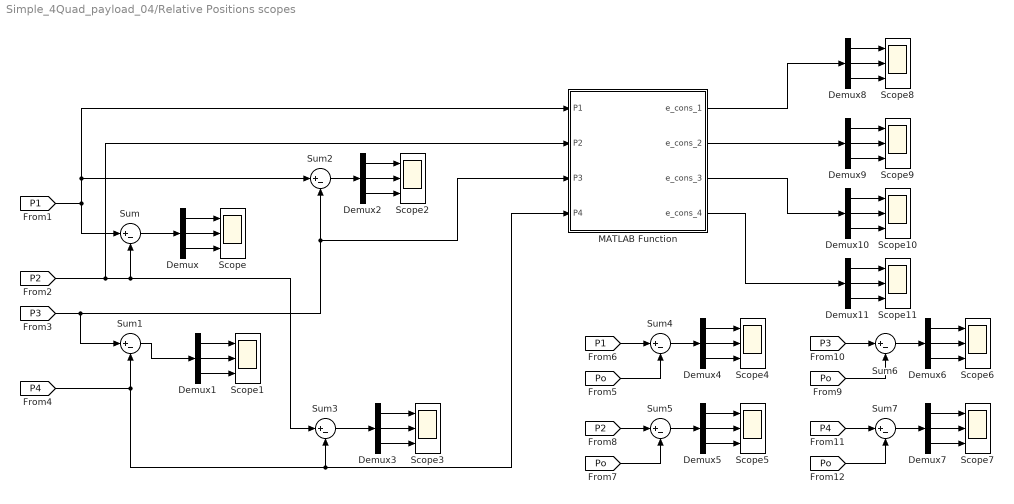
== system Simple_4Quad_payload_04/Relative Positions scopes ==
  Demux{,1..11} (12 alike) : Demux  Outputs=3
  MATLAB Function : MATLAB Function  TreatAsAtomicUnit=on
  Scope{,1..11} (12 alike) : Scope  NumInputPorts=3
  Sum{,1..7} (8 alike) : Sum  Inputs=|+-
  wires:
  Demux/3 -> Scope/3
  Demux/1 -> Scope/1
  Demux/2 -> Scope/2
  Sum/1 -> Demux/1
  Sum1/1 -> Demux1/1
  Demux1/2 -> Scope1/2
  Demux1/1 -> Scope1/1
  Demux1/3 -> Scope1/3
  Sum2/1 -> Demux2/1
  [P3] -> MATLAB Function/3(P3), Sum2/2, Sum1/1
  [P1] -> Sum/1, Sum2/1, MATLAB Function/1(P1)
  Demux2/2 -> Scope2/2
  Demux2/1 -> Scope2/1
  Demux2/3 -> Scope2/3
  Demux3/3 -> Scope3/3
  Demux3/1 -> Scope3/1
  Demux3/2 -> Scope3/2
  [P2] -> MATLAB Function/2(P2), Sum/2, Sum3/1
  [P4] -> Sum3/2, MATLAB Function/4(P4), Sum1/2
  Sum3/1 -> Demux3/1
  Demux4/3 -> Scope4/3
  Demux4/1 -> Scope4/1
  Demux4/2 -> Scope4/2
  Sum4/1 -> Demux4/1
  Sum5/1 -> Demux5/1
  Demux5/2 -> Scope5/2
  Demux5/1 -> Scope5/1
  Demux5/3 -> Scope5/3
  Demux6/3 -> Scope6/3
  Demux6/1 -> Scope6/1
  Demux6/2 -> Scope6/2
  Sum6/1 -> Demux6/1
  Sum7/1 -> Demux7/1
  Demux7/2 -> Scope7/2
  Demux7/1 -> Scope7/1
  Demux7/3 -> Scope7/3
  [Po] -> Sum4/2
  [P1] -> Sum4/1
  [P2] -> Sum5/1
  [Po] -> Sum5/2
  [P3] -> Sum6/1
  [Po] -> Sum6/2
  [P4] -> Sum7/1
  [Po] -> Sum7/2
  Demux8/2 -> Scope8/2
  Demux8/1 -> Scope8/1
  Demux8/3 -> Scope8/3
  MATLAB Function/1(e_cons_1) -> Demux8/1
  Demux9/3 -> Scope9/3
  Demux9/1 -> Scope9/1
  Demux9/2 -> Scope9/2
  MATLAB Function/2(e_cons_2) -> Demux9/1
  Demux10/2 -> Scope10/2
  Demux10/1 -> Scope10/1
  Demux10/3 -> Scope10/3
  MATLAB Function/3(e_cons_3) -> Demux10/1
  Demux11/3 -> Scope11/3
  Demux11/1 -> Scope11/1
  Demux11/2 -> Scope11/2
  MATLAB Function/4(e_cons_4) -> Demux11/1

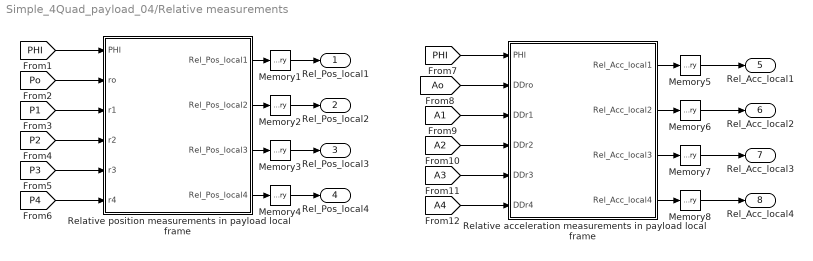
== system Simple_4Quad_payload_04/Relative measurements ==
  Memory{1..8} (8 alike) : Memory  InitialCondition=zeros(3,1)
  Relative acceleration measurements in payload local frame : MATLAB Function  TreatAsAtomicUnit=on
  Relative position measurements in payload local frame : MATLAB Function  TreatAsAtomicUnit=on
  Rel_Pos_local1 : Outport
  Rel_Pos_local2 : Outport  Port=2
  Rel_Pos_local3 : Outport  Port=3
  Rel_Pos_local4 : Outport  Port=4
  Rel_Acc_local1 : Outport  Port=5
  Rel_Acc_local2 : Outport  Port=6
  Rel_Acc_local3 : Outport  Port=7
  Rel_Acc_local4 : Outport  Port=8
  wires:
  [PHI] -> Relative position measurements in payload local frame/1(PHI)
  [Po] -> Relative position measurements in payload local frame/2(ro)
  [P1] -> Relative position measurements in payload local frame/3(r1)
  [P2] -> Relative position measurements in payload local frame/4(r2)
  [P3] -> Relative position measurements in payload local frame/5(r3)
  [P4] -> Relative position measurements in payload local frame/6(r4)
  Relative position measurements in payload local frame/1(Rel_Pos_local1) -> Memory1/1
  Relative position measurements in payload local frame/2(Rel_Pos_local2) -> Memory2/1
  Relative position measurements in payload local frame/3(Rel_Pos_local3) -> Memory3/1
  Relative position measurements in payload local frame/4(Rel_Pos_local4) -> Memory4/1
  Relative acceleration measurements in payload local frame/4(Rel_Acc_local4) -> Memory8/1
  Relative acceleration measurements in payload local frame/3(Rel_Acc_local3) -> Memory7/1
  Relative acceleration measurements in payload local frame/2(Rel_Acc_local2) -> Memory6/1
  Relative acceleration measurements in payload local frame/1(Rel_Acc_local1) -> Memory5/1
  [A4] -> Relative acceleration measurements in payload local frame/6(DDr4)
  [A3] -> Relative acceleration measurements in payload local frame/5(DDr3)
  [A2] -> Relative acceleration measurements in payload local frame/4(DDr2)
  [A1] -> Relative acceleration measurements in payload local frame/3(DDr1)
  [Ao] -> Relative acceleration measurements in payload local frame/2(DDro)
  [PHI] -> Relative acceleration measurements in payload local frame/1(PHI)
  Memory1/1 -> Rel_Pos_local1/1
  Memory2/1 -> Rel_Pos_local2/1
  Memory3/1 -> Rel_Pos_local3/1
  Memory4/1 -> Rel_Pos_local4/1
  Memory5/1 -> Rel_Acc_local1/1
  Memory6/1 -> Rel_Acc_local2/1
  Memory7/1 -> Rel_Acc_local3/1
  Memory8/1 -> Rel_Acc_local4/1

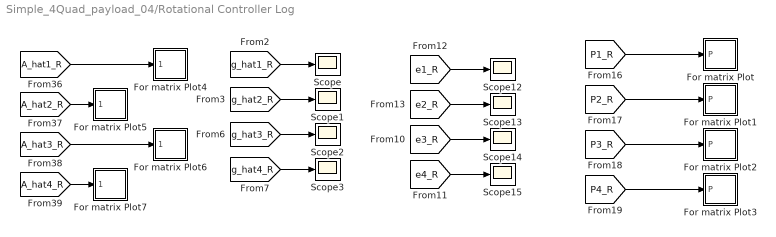
== system Simple_4Quad_payload_04/Rotational Controller Log ==
  For matrix Plot : Subsystem
  For matrix Plot1 : Subsystem
  For matrix Plot2 : Subsystem
  For matrix Plot3 : Subsystem
  For matrix Plot4 : Subsystem
  For matrix Plot5 : Subsystem
  For matrix Plot6 : Subsystem
  For matrix Plot7 : Subsystem
  Scope{,1..3,12..15} (8 alike) : Scope
  wires:
  [g_hat1_R] -> Scope/1
  [g_hat3_R] -> Scope2/1
  [g_hat2_R] -> Scope1/1
  [g_hat4_R] -> Scope3/1
  [e2_R] -> Scope13/1
  [P1_R] -> For matrix Plot/1(P)
  [e4_R] -> Scope15/1
  [P4_R] -> For matrix Plot3/1(P)
  [e3_R] -> Scope14/1
  [P3_R] -> For matrix Plot2/1(P)
  [e1_R] -> Scope12/1
  [P2_R] -> For matrix Plot1/1(P)
  [A_hat4_R] -> For matrix Plot7/1(A_hat)
  [A_hat2_R] -> For matrix Plot5/1(A_hat)
  [A_hat1_R] -> For matrix Plot4/1(A_hat)
  [A_hat3_R] -> For matrix Plot6/1(A_hat)

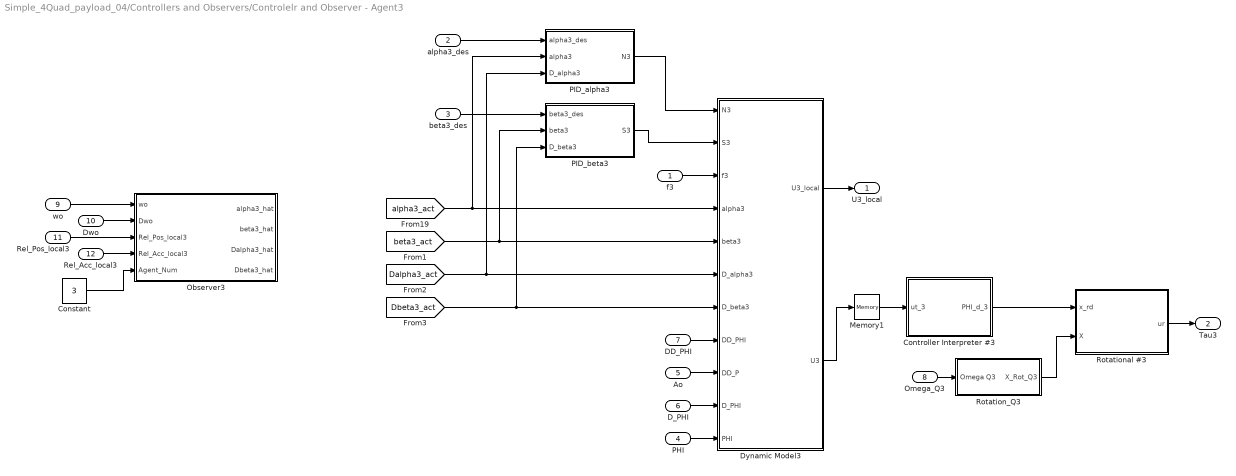
== system Simple_4Quad_payload_04/Controllers and Observers/Controlelr and Observer - Agent3 ==
  f3 : Inport
  alpha3_des : Inport  Port=2
  beta3_des : Inport  Port=3
  PHI : Inport  Port=4
  Ao : Inport  Port=5
  D_PHI : Inport  Port=6
  DD_PHI : Inport  Port=7
  Omega_Q3 : Inport  Port=8
  wo : Inport  Port=9
  Dwo : Inport  Port=10
  Rel_Pos_local3 : Inport  Port=11
  Rel_Acc_local3 : Inport  Port=12
  Constant : Constant  Value=3
  Controller Interpreter #3 : MATLAB Function  TreatAsAtomicUnit=on
  Dynamic Model3 : MATLAB Function  TreatAsAtomicUnit=on
  Memory1 : Memory  InitialCondition=zeros(3,1)
  Observer3 : Subsystem
  PID_alpha3 : Subsystem
  PID_beta3 : Subsystem
  Rotation_Q3 : Subsystem
  Rotational #3 : Subsystem
  U3_local : Outport
  Tau3 : Outport  Port=2
  wires:
  PID_alpha3/1(N3) -> Dynamic Model3/1(N3)
  PID_beta3/1(S3) -> Dynamic Model3/2(S3)
  f3/1 -> Dynamic Model3/3(f3)
  Memory1/1 -> Controller Interpreter #3/1(ut_3)
  alpha3_des/1 -> PID_alpha3/1(alpha3_des)
  Dynamic Model3/2(U3) -> Memory1/1
  DD_PHI/1 -> Dynamic Model3/8(DD_PHI)
  D_PHI/1 -> Dynamic Model3/10(D_PHI)
  Ao/1 -> Dynamic Model3/9(DD_P)
  PHI/1 -> Dynamic Model3/11(PHI)
  beta3_des/1 -> PID_beta3/1(beta3_des)
  Dynamic Model3/1(U3_local) -> U3_local/1
  Controller Interpreter #3/1(PHI_d_3) -> Rotational #3/1(x_rd)
  Rotational #3/1(ur) -> Tau3/1
  Omega_Q3/1 -> Rotation_Q3/1(Omega Q3)
  Rotation_Q3/1(X_Rot_Q3) -> Rotational #3/2(X)
  wo/1 -> Observer3/1(wo)
  Dwo/1 -> Observer3/2(Dwo)
  Rel_Pos_local3/1 -> Observer3/3(Rel_Pos_local3)
  Rel_Acc_local3/1 -> Observer3/4(Rel_Acc_local3)
  [alpha3_act] -> PID_alpha3/2(alpha3), Dynamic Model3/4(alpha3)
  [beta3_act] -> PID_beta3/2(beta3), Dynamic Model3/5(beta3)
  [Dalpha3_act] -> PID_alpha3/3(D_alpha3), Dynamic Model3/6(D_alpha3)
  [Dbeta3_act] -> PID_beta3/3(D_beta3), Dynamic Model3/7(D_beta3)
  Constant/1 -> Observer3/5(Agent_Num)

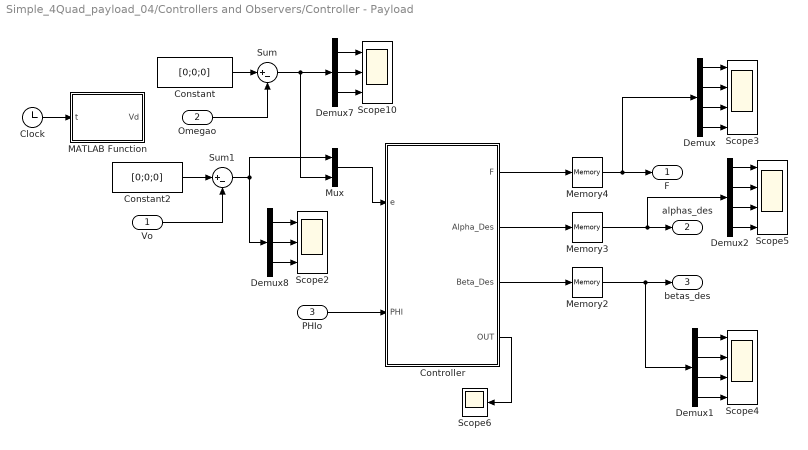
== system Simple_4Quad_payload_04/Controllers and Observers/Controller - Payload ==
  Vo : Inport
  Omegao : Inport  Port=2
  PHIo : Inport  Port=3
  Clock : Clock
  Constant : Constant  Value=[0;0;0]
  Constant2 : Constant  Value=[0;0;0]
  Controller : MATLAB Function  TreatAsAtomicUnit=on
  Demux : Demux
  Demux1 : Demux
  Demux2 : Demux
  Demux7 : Demux  Outputs=3
  Demux8 : Demux  Outputs=3
  MATLAB Function : MATLAB Function  TreatAsAtomicUnit=on
  Memory2 : Memory  InitialCondition=[0;pi;pi/2;-pi/2]
  Memory3 : Memory  InitialCondition=pi/2*ones(4,1)
  Memory4 : Memory  InitialCondition=zeros(4,1)
  Mux : Mux  Inputs=2
  Scope10 : Scope  NumInputPorts=3
  Scope2 : Scope  NumInputPorts=3
  Scope3 : Scope  NumInputPorts=4
  Scope4 : Scope  NumInputPorts=4
  Scope5 : Scope  NumInputPorts=4
  Scope6 : Scope
  Sum : Sum  Inputs=|+-
  Sum1 : Sum  Inputs=|+-
  F : Outport
  alphas_des : Outport  Port=2
  betas_des : Outport  Port=3
  wires:
  Constant/1 -> Sum/1
  Constant2/1 -> Sum1/1
  Controller/4(OUT) -> Scope6/1
  Mux/1 -> Controller/1(e)
  Controller/1(F) -> Memory4/1
  Controller/2(Alpha_Des) -> Memory3/1
  Demux/1 -> Scope3/1
  Demux/2 -> Scope3/2
  Demux/3 -> Scope3/3
  Demux/4 -> Scope3/4
  Demux1/4 -> Scope4/4
  Demux1/3 -> Scope4/3
  Demux1/2 -> Scope4/2
  Demux1/1 -> Scope4/1
  Controller/3(Beta_Des) -> Memory2/1
  Demux2/1 -> Scope5/1
  Demux2/2 -> Scope5/2
  Demux2/3 -> Scope5/3
  Demux2/4 -> Scope5/4
  Sum1/1 -> Demux8/1, Mux/1
  Demux7/3 -> Scope10/3
  Demux7/2 -> Scope10/2
  Demux7/1 -> Scope10/1
  Demux8/1 -> Scope2/1
  Demux8/2 -> Scope2/2
  Demux8/3 -> Scope2/3
  Sum/1 -> Demux7/1, Mux/2
  Memory2/1 -> betas_des/1, Demux1/1
  Memory3/1 -> Demux2/1, alphas_des/1
  Memory4/1 -> Demux/1, F/1
  Clock/1 -> MATLAB Function/1(t)
  Vo/1 -> Sum1/2
  Omegao/1 -> Sum/2
  PHIo/1 -> Controller/2(PHI)

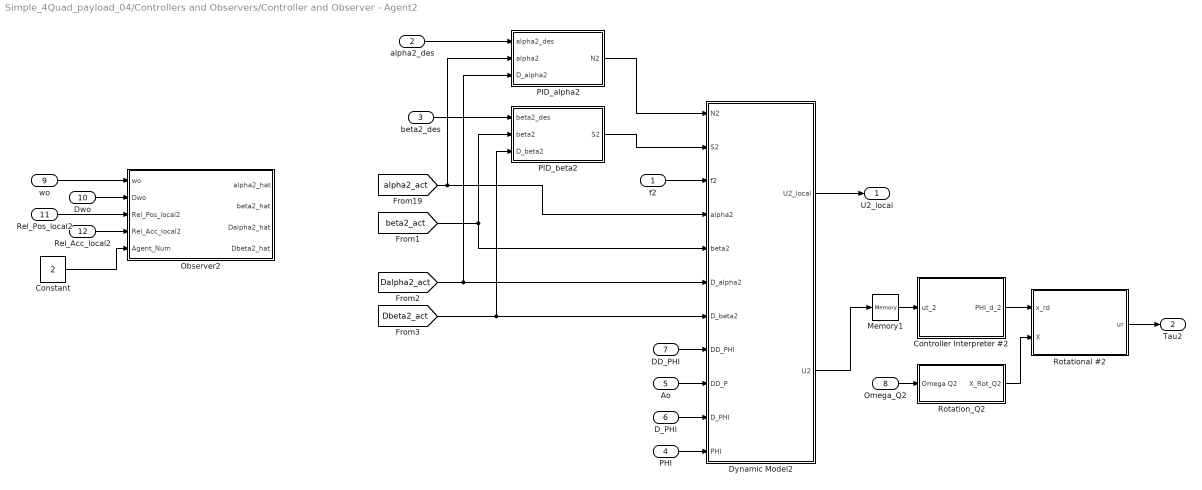
== system Simple_4Quad_payload_04/Controllers and Observers/Controller and Observer - Agent2 ==
  f2 : Inport
  alpha2_des : Inport  Port=2
  beta2_des : Inport  Port=3
  PHI : Inport  Port=4
  Ao : Inport  Port=5
  D_PHI : Inport  Port=6
  DD_PHI : Inport  Port=7
  Omega_Q2 : Inport  Port=8
  wo : Inport  Port=9
  Dwo : Inport  Port=10
  Rel_Pos_local2 : Inport  Port=11
  Rel_Acc_local2 : Inport  Port=12
  Constant : Constant  Value=2
  Controller Interpreter #2 : MATLAB Function  TreatAsAtomicUnit=on
  Dynamic Model2 : MATLAB Function  TreatAsAtomicUnit=on
  Memory1 : Memory  InitialCondition=zeros(3,1)
  Observer2 : Subsystem
  PID_alpha2 : Subsystem
  PID_beta2 : Subsystem
  Rotation_Q2 : Subsystem
  Rotational #2 : Subsystem
  U2_local : Outport
  Tau2 : Outport  Port=2
  wires:
  Memory1/1 -> Controller Interpreter #2/1(ut_2)
  alpha2_des/1 -> PID_alpha2/1(alpha2_des)
  Dynamic Model2/2(U2) -> Memory1/1
  f2/1 -> Dynamic Model2/3(f2)
  DD_PHI/1 -> Dynamic Model2/8(DD_PHI)
  D_PHI/1 -> Dynamic Model2/10(D_PHI)
  Ao/1 -> Dynamic Model2/9(DD_P)
  PHI/1 -> Dynamic Model2/11(PHI)
  PID_alpha2/1(N2) -> Dynamic Model2/1(N2)
  beta2_des/1 -> PID_beta2/1(beta2_des)
  PID_beta2/1(S2) -> Dynamic Model2/2(S2)
  Dynamic Model2/1(U2_local) -> U2_local/1
  Controller Interpreter #2/1(PHI_d_2) -> Rotational #2/1(x_rd)
  Rotational #2/1(ur) -> Tau2/1
  Omega_Q2/1 -> Rotation_Q2/1(Omega Q2)
  Rotation_Q2/1(X_Rot_Q2) -> Rotational #2/2(X)
  [alpha2_act] -> PID_alpha2/2(alpha2), Dynamic Model2/4(alpha2)
  [Dalpha2_act] -> PID_alpha2/3(D_alpha2), Dynamic Model2/6(D_alpha2)
  [beta2_act] -> Dynamic Model2/5(beta2), PID_beta2/2(beta2)
  [Dbeta2_act] -> PID_beta2/3(D_beta2), Dynamic Model2/7(D_beta2)
  wo/1 -> Observer2/1(wo)
  Dwo/1 -> Observer2/2(Dwo)
  Rel_Pos_local2/1 -> Observer2/3(Rel_Pos_local2)
  Rel_Acc_local2/1 -> Observer2/4(Rel_Acc_local2)
  Constant/1 -> Observer2/5(Agent_Num)

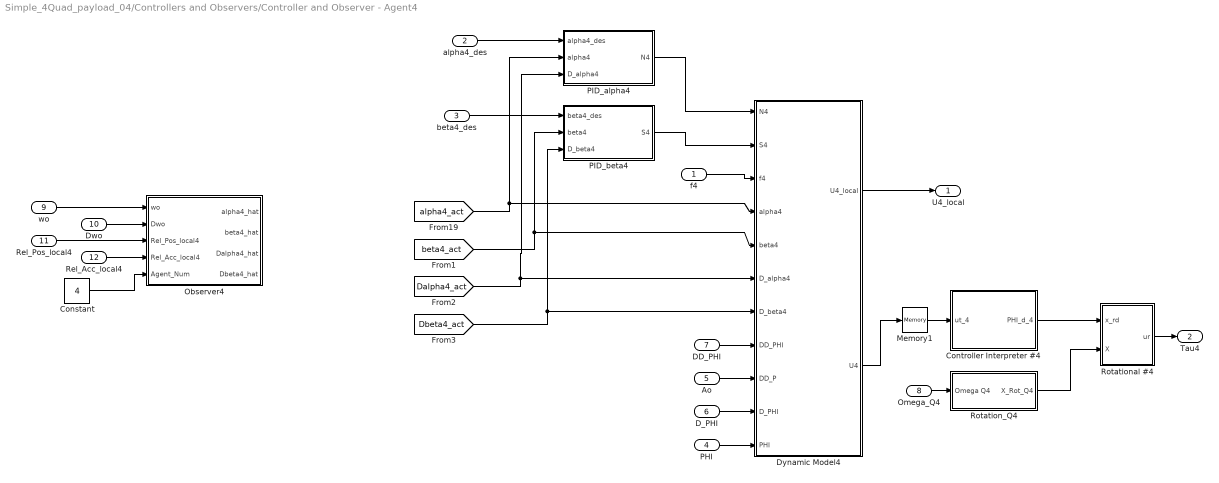
== system Simple_4Quad_payload_04/Controllers and Observers/Controller and Observer - Agent4 ==
  f4 : Inport
  alpha4_des : Inport  Port=2
  beta4_des : Inport  Port=3
  PHI : Inport  Port=4
  Ao : Inport  Port=5
  D_PHI : Inport  Port=6
  DD_PHI : Inport  Port=7
  Omega_Q4 : Inport  Port=8
  wo : Inport  Port=9
  Dwo : Inport  Port=10
  Rel_Pos_local4 : Inport  Port=11
  Rel_Acc_local4 : Inport  Port=12
  Constant : Constant  Value=4
  Controller Interpreter #4 : MATLAB Function  TreatAsAtomicUnit=on
  Dynamic Model4 : MATLAB Function  TreatAsAtomicUnit=on
  Memory1 : Memory  InitialCondition=zeros(3,1)
  Observer4 : Subsystem
  PID_alpha4 : Subsystem
  PID_beta4 : Subsystem
  Rotation_Q4 : Subsystem
  Rotational #4 : Subsystem
  U4_local : Outport
  Tau4 : Outport  Port=2
  wires:
  Memory1/1 -> Controller Interpreter #4/1(ut_4)
  PID_beta4/1(S4) -> Dynamic Model4/2(S4)
  beta4_des/1 -> PID_beta4/1(beta4_des)
  PID_alpha4/1(N4) -> Dynamic Model4/1(N4)
  PHI/1 -> Dynamic Model4/11(PHI)
  Ao/1 -> Dynamic Model4/9(DD_P)
  D_PHI/1 -> Dynamic Model4/10(D_PHI)
  DD_PHI/1 -> Dynamic Model4/8(DD_PHI)
  f4/1 -> Dynamic Model4/3(f4)
  Dynamic Model4/2(U4) -> Memory1/1
  alpha4_des/1 -> PID_alpha4/1(alpha4_des)
  Dynamic Model4/1(U4_local) -> U4_local/1
  Controller Interpreter #4/1(PHI_d_4) -> Rotational #4/1(x_rd)
  Rotational #4/1(ur) -> Tau4/1
  Omega_Q4/1 -> Rotation_Q4/1(Omega Q4)
  Rotation_Q4/1(X_Rot_Q4) -> Rotational #4/2(X)
  Rel_Pos_local4/1 -> Observer4/3(Rel_Pos_local4)
  Dwo/1 -> Observer4/2(Dwo)
  wo/1 -> Observer4/1(wo)
  Rel_Acc_local4/1 -> Observer4/4(Rel_Acc_local4)
  [alpha4_act] -> Dynamic Model4/4(alpha4), PID_alpha4/2(alpha4)
  [beta4_act] -> Dynamic Model4/5(beta4), PID_beta4/2(beta4)
  [Dalpha4_act] -> PID_alpha4/3(D_alpha4), Dynamic Model4/6(D_alpha4)
  [Dbeta4_act] -> PID_beta4/3(D_beta4), Dynamic Model4/7(D_beta4)
  Constant/1 -> Observer4/5(Agent_Num)

== system Simple_4Quad_payload_04/Controllers and Observers/Cotnroller and Observer - Agent1  ==
  f1 : Inport
  alpha1_des : Inport  Port=2
  beta1_des : Inport  Port=3
  PHI : Inport  Port=4
  Ao : Inport  Port=5
  D_PHI : Inport  Port=6
  DD_PHI : Inport  Port=7
  Omega_Q1 : Inport  Port=8
  wo : Inport  Port=9
  Dwo : Inport  Port=10
  Rel_Pos_local1 : Inport  Port=11
  Rel_Acc_local1 : Inport  Port=12
  Constant : Constant
  Controller Interpreter #1 : MATLAB Function  TreatAsAtomicUnit=on
  Dynamic Model1 : MATLAB Function  TreatAsAtomicUnit=on
  Memory1 : Memory  InitialCondition=zeros(3,1)
  Observer1 : Subsystem
  PID_alpha1 : Subsystem
  PID_beta1 : Subsystem
  Rotation_Q1 : Subsystem
  Rotational #1 : Subsystem
  U1_local : Outport
  Tau1 : Outport  Port=2
  wires:
  PID_alpha1/1(N1) -> Dynamic Model1/1(N1)
  PID_beta1/1(S1) -> Dynamic Model1/2(S1)
  f1/1 -> Dynamic Model1/3(f1)
  Memory1/1 -> Controller Interpreter #1/1(ut_1)
  beta1_des/1 -> PID_beta1/1(beta1_des)
  PHI/1 -> Dynamic Model1/11(PHI)
  Ao/1 -> Dynamic Model1/9(DD_P)
  D_PHI/1 -> Dynamic Model1/10(D_PHI)
  DD_PHI/1 -> Dynamic Model1/8(DD_PHI)
  Dynamic Model1/2(U1) -> Memory1/1
  alpha1_des/1 -> PID_alpha1/1(alpha1_des)
  Dynamic Model1/1(U1_local) -> U1_local/1
  Controller Interpreter #1/1(PHI_d_1) -> Rotational #1/1(x_rd)
  Rotational #1/1(ur1) -> Tau1/1
  Omega_Q1/1 -> Rotation_Q1/1(Omega Q1)
  Rotation_Q1/1(X_Rot_Q1) -> Rotational #1/2(X)
  [alpha1_act] -> Dynamic Model1/4(alpha1), PID_alpha1/2(alpha1)
  [Dalpha1_act] -> PID_alpha1/3(D_alpha1), Dynamic Model1/6(D_alpha1)
  [beta1_act] -> PID_beta1/2(beta1), Dynamic Model1/5(beta1)
  [Dbeta1_act] -> PID_beta1/3(D_beta1), Dynamic Model1/7(D_beta1)
  wo/1 -> Observer1/1(wo)
  Dwo/1 -> Observer1/2(Dwo)
  Rel_Pos_local1/1 -> Observer1/3(Rel_Pos_local1)
  Rel_Acc_local1/1 -> Observer1/4(Rel_Acc_local1)
  Constant/1 -> Observer1/5(Agent_Num)

== system Simple_4Quad_payload_04/Rotational Controller Log/For matrix Plot ==
  P : Inport
  MATLAB Function : MATLAB Function  TreatAsAtomicUnit=on
  To Workspace : ToWorkspace  VariableName=P1_R  SaveFormat=Structure With Time  SampleTime=-1
  wires:
  MATLAB Function/1(y) -> To Workspace/1
  P/1 -> MATLAB Function/1(u)

== system Simple_4Quad_payload_04/Rotational Controller Log/For matrix Plot1 ==
  P : Inport
  MATLAB Function : MATLAB Function  TreatAsAtomicUnit=on
  To Workspace : ToWorkspace  VariableName=P2_R  SaveFormat=Structure With Time  SampleTime=-1
  wires:
  P/1 -> MATLAB Function/1(u)
  MATLAB Function/1(y) -> To Workspace/1

== system Simple_4Quad_payload_04/Rotational Controller Log/For matrix Plot2 ==
  P : Inport
  MATLAB Function : MATLAB Function  TreatAsAtomicUnit=on
  To Workspace : ToWorkspace  VariableName=P3_R  SaveFormat=Structure With Time  SampleTime=-1
  wires:
  P/1 -> MATLAB Function/1(u)
  MATLAB Function/1(y) -> To Workspace/1

== system Simple_4Quad_payload_04/Rotational Controller Log/For matrix Plot3 ==
  P : Inport
  MATLAB Function : MATLAB Function  TreatAsAtomicUnit=on
  To Workspace : ToWorkspace  VariableName=P4_R  SaveFormat=Structure With Time  SampleTime=-1
  wires:
  MATLAB Function/1(y) -> To Workspace/1
  P/1 -> MATLAB Function/1(u)

== system Simple_4Quad_payload_04/Rotational Controller Log/For matrix Plot4 ==
  A_hat : Inport
  MATLAB Function : MATLAB Function  TreatAsAtomicUnit=on
  To Workspace : ToWorkspace  VariableName=A_hat1_R  SaveFormat=Structure With Time  SampleTime=-1
  wires:
  A_hat/1 -> MATLAB Function/1(u)
  MATLAB Function/1(y) -> To Workspace/1

== system Simple_4Quad_payload_04/Rotational Controller Log/For matrix Plot5 ==
  A_hat : Inport
  MATLAB Function : MATLAB Function  TreatAsAtomicUnit=on
  To Workspace : ToWorkspace  VariableName=A_hat2_R  SaveFormat=Structure With Time  SampleTime=-1
  wires:
  MATLAB Function/1(y) -> To Workspace/1
  A_hat/1 -> MATLAB Function/1(u)

== system Simple_4Quad_payload_04/Rotational Controller Log/For matrix Plot6 ==
  A_hat : Inport
  MATLAB Function : MATLAB Function  TreatAsAtomicUnit=on
  To Workspace : ToWorkspace  VariableName=A_hat3_R  SaveFormat=Structure With Time  SampleTime=-1
  wires:
  A_hat/1 -> MATLAB Function/1(u)
  MATLAB Function/1(y) -> To Workspace/1

== system Simple_4Quad_payload_04/Rotational Controller Log/For matrix Plot7 ==
  A_hat : Inport
  MATLAB Function : MATLAB Function  TreatAsAtomicUnit=on
  To Workspace : ToWorkspace  VariableName=A_hat4_R  SaveFormat=Structure With Time  SampleTime=-1
  wires:
  MATLAB Function/1(y) -> To Workspace/1
  A_hat/1 -> MATLAB Function/1(u)

== system Simple_4Quad_payload_04/Controllers and Observers/Controlelr and Observer - Agent3/Observer3 ==
  wo : Inport
  Dwo : Inport  Port=2
  Rel_Pos_local3 : Inport  Port=3
  Rel_Acc_local3 : Inport  Port=4
  Agent_Num : Inport  Port=5
  Integrator : Integrator  InitialCondition=eye(6)
  Integrator1 : Integrator  InitialCondition=[0;0;1;0;0;0]
  Kalman_Filter3 : MATLAB Function  TreatAsAtomicUnit=on
  Observer_Finalization3 : MATLAB Function  TreatAsAtomicUnit=on
  alpha3_hat : Outport
  beta3_hat : Outport  Port=2
  Dalpha3_hat : Outport  Port=3
  Dbeta3_hat : Outport  Port=4
  tag scope: Dalpha_hat3=global, Dbeta_hat3=global, alpha_hat3=global, beta_hat3=global
  wires:
  Kalman_Filter3/1(DP_ob) -> Integrator/1
  Kalman_Filter3/2(Dxhat_ob) -> Integrator1/1
  Integrator/1 -> Kalman_Filter3/1(P_ob)
  Integrator1/1 -> Observer_Finalization3/1(xhati), Kalman_Filter3/2(xhat_ob)
  wo/1 -> Kalman_Filter3/3(wo)
  Dwo/1 -> Kalman_Filter3/4(Dwo)
  Observer_Finalization3/1(alphai_hat) -> [alpha_hat3], alpha3_hat/1
  Observer_Finalization3/2(betai_hat) -> [beta_hat3], beta3_hat/1
  Observer_Finalization3/3(Dalphai_hat) -> [Dalpha_hat3], Dalpha3_hat/1
  Observer_Finalization3/4(Dbetai_hat) -> [Dbeta_hat3], Dbeta3_hat/1
  Rel_Pos_local3/1 -> Kalman_Filter3/5(Rel_Posi_local)
  Rel_Acc_local3/1 -> Kalman_Filter3/6(Rel_Acci_local)
  Agent_Num/1 -> Kalman_Filter3/7(Agent_Num)
